simulink model "Modified_singlephasevienna"  (R2024a)
settings: Solver=VariableStepAuto  StartTime=0.0  StopTime=5  RelTol=1e-3
libraries: spsVoltageMeasurementLib x11, spsDiodeLib x10, spsCurrentMeasurementLib x8, spsSeriesRLCBranchLib x7, spsMosfetLib x4, spsIdealSwitchLib x2, slpidlib x2, spsVariableResistorLib x2, spsACVoltageSourceLib x1, simulink_extras x1, spsIGBTLib x1, spsLinearTransformerLib x1
settings Model: Creator=DELL  LastModifiedBy=DELL

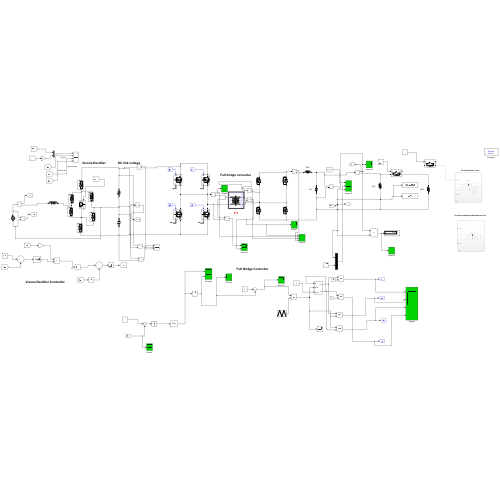
[thumbnail: Simulink's stored preview of the top-level diagram]
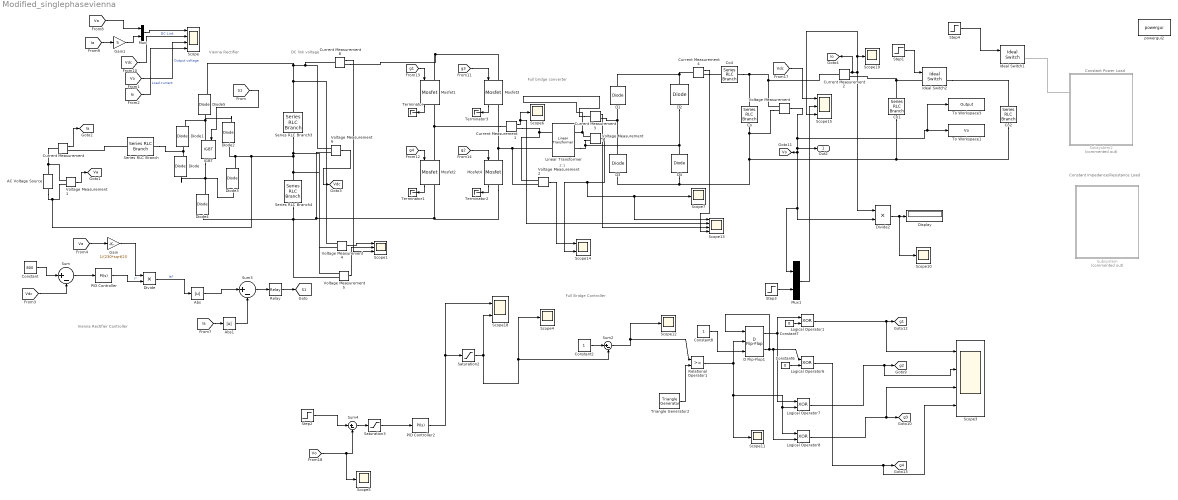
== system Modified_singlephasevienna ==
  note: Constant Power Load
  note: 2:1
  note: Full bridge converter
  note: Constant Impedance/Resistance Load
  note: Vienna Rectifier
  note: Vienna Rectifier Controller
  note: Full Bridge Controller
  note: DC link voltage
  AC Voltage Source : spsACVoltageSourceLib/AC Voltage Source  Amplitude=325  Phase=0  Frequency=50  SampleTime=0  Measurements=None  BusType=PV  Pref=10e3  Qref=0  Qmin=-inf  Qmax=+inf
  Abs : Abs  SaturateOnIntegerOverflow=off
  Abs1 : Abs  SaturateOnIntegerOverflow=off
  Co : spsSeriesRLCBranchLib/Series RLC Branch  LConnTagsString=__new0  RConnTagsString=__new0  BranchType=C  Resistance=1e-4  Inductance=200e-6  SetiL0=off  InitialCurrent=0  Capacitance=2000e-6  Setx0=off  InitialVoltage=24  Measurements=None
  Co1 : spsSeriesRLCBranchLib/Series RLC Branch  LConnTagsString=__new0  RConnTagsString=__new0  BranchType=R  Resistance=0.52  Inductance=200e-6  SetiL0=off  InitialCurrent=0  Capacitance=1000e-6  Setx0=off  InitialVoltage=24  Measurements=None
  Co2 : spsSeriesRLCBranchLib/Series RLC Branch  LConnTagsString=__new0  RConnTagsString=__new0  BranchType=R  Resistance=0.52  Inductance=200e-6  SetiL0=off  InitialCurrent=0  Capacitance=1000e-6  Setx0=off  InitialVoltage=24  Measurements=None
  Co4 : spsSeriesRLCBranchLib/Series RLC Branch  LConnTagsString=__new0  RConnTagsString=__new0  BranchType=L  Resistance=1e-4  Inductance=.01  SetiL0=off  InitialCurrent=0  Capacitance=1000e-6  Setx0=off  InitialVoltage=24  Measurements=None
  Constant : Constant  Value=800
  Constant2 : Constant
  Constant6 : Constant  Value=0
  Constant7 : Constant  Value=0
  Constant8 : Constant
  Current Measurement{,1..4,8} (6 alike) : spsCurrentMeasurementLib/Current Measurement  PhasorSimulation=off  OutputType=Complex  PSBequivalent=0
  D Flip-Flop1 : simulink_extras/Flip Flops/D Flip-Flop
  D{1..4} (4 alike) : spsDiodeLib/Diode  Ron=1e-3  Lon=0  Vf=0.5  IC=0  UseSnubber=off  Rs=1e6  Cs=inf  Measurements=off
  Diode{,1..5} (6 alike) : spsDiodeLib/Diode  Ron=0.001  Lon=0  Vf=0.8  IC=0  UseSnubber=0  Rs=500  Cs=250e-9  Measurements=on
  Display : Display
  Divide : Product  Inputs=**
  Divide2 : Product  Inputs=**
  Gain : Gain  Gain=1/(230*sqrt(2))
  Gain1 : Gain  Gain=5
  IGBT : spsIGBTLib/IGBT  Ron=0.001  Lon=0  Vf=1  Tf=1e-6  Tt=2e-6  IC=0  Rs=1e5  Cs=inf  Measurements=on
  Ideal Switch1 : spsIdealSwitchLib/Ideal Switch  Ron=0.001  Lon=0  IC=0  Rs=1e5  Cs=inf  Measurements=on
  Ideal Switch2 : spsIdealSwitchLib/Ideal Switch  Ron=0.001  Lon=0  IC=0  Rs=1e5  Cs=inf  Measurements=on
  Linear Transformer : spsLinearTransformerLib/Linear Transformer  UNITS=SI  NominalPower=[3000 10e3 ]  winding1="[200   1e-2  100e-6]"  winding2="[100  1e-2  1.36e-6 ]"  ThreeWindings=off  winding3=[50 1e-2 1.36e-6]  RmLm=[10e3 0.01]  Measurements=None  DataType=on
  Logical Operator{1,6..8} (4 alike) : Logic  Operator=XOR  AllPortsSameDT=off  OutDataTypeStr=boolean
  Mosfet{1..4} (4 alike) : spsMosfetLib/Mosfet  Ron=1e-3  Lon=0  Rd=1e-3  Vfd=0  IC=0  Rs=1e6  Cs=inf  Measurements=on
  Mux : Mux  Inputs=2
  Mux1 : Mux  Inputs=2
  PID Controller : slpidlib/PID Controller  Controller=PI  Form=Parallel  TimeDomain=Continuous-time  UseExternalTs=off  SampleTime=50e-6  IntegratorMethod=Forward Euler  FilterMethod=Forward Euler  ControllerParametersSource=internal  P=5  I=100  UseKiTs=off  D=0  UseExternalDerivativeSource=off  N=100  UseFilter=on  TunerSelectOption=Transfer Function Based (PID Tuner App)  InitialConditionSource=internal  InitialConditionForIntegrator=0  InitialConditionForFilter=0  DifferentiatorICPrevScaledInput=0  ExternalReset=none  TrackingMode=off  Kt=1  LimitOutput=on  SatLimitsSource=internal  UpperSaturationLimit=30  LowerSaturationLimit=0  LinearizeAsGain=on  AntiWindupMode=none  Kb=1  LimitIntegrator=off  UpperIntegratorSaturationLimit=inf  LowerIntegratorSaturationLimit=-inf  POutMin=[]  POutMax=[]  IOutMin=[]  IOutMax=[]  DOutMin=[]  DOutMax=[]  NOutMin=[]  NOutMax=[]  SumOutMin=[]  SumOutMax=[]  SaturationOutMin=[]  SaturationOutMax=[]  PParamMin=[]  PParamMax=[]  IParamMin=[]  IParamMax=[]  DParamMin=[]  DParamMax=[]  NParamMin=[]  NParamMax=[]  KbParamMin=[]  KbParamMax=[]  KtParamMin=[]  KtParamMax=[]  KbOutMin=[]  KbOutMax=[]  KtOutMin=[]  KtOutMax=[]  IntegratorOutMin=[]  IntegratorOutMax=[]  FilterOutMin=[]  FilterOutMax=[]  SumI1OutMin=[]  SumI1OutMax=[]  SumI2OutMin=[]  SumI2OutMax=[]  SumI3OutMin=[]  SumI3OutMax=[]  SumI4OutMin=[]  SumI4OutMax=[]  SumDOutMin=[]  SumDOutMax=[]  DifferentiatorOutMin=[]  DifferentiatorOutMax=[]  FilterDiffOutCoefMin=[]  FilterDiffOutCoefMax=[]  ReciprocalOutMin=[]  ReciprocalOutMax=[]  SumDenOutMin=[]  SumDenOutMax=[]  SumNumOutMin=[]  SumNumOutMax=[]  DivideOutMin=[]  DivideOutMax=[]  UdiffTsProdOutMin=[]  UdiffTsProdOutMax=[]  NTsProdOutMin=[]  NTsProdOutMax=[]  UintegralTsProdOutMin=[]  UintegralTsProdOutMax=[]  UngainTsProdOutMin=[]  UngainTsProdOutMax=[]  ClampingZeroOutDataTypeStr=Inherit: Inherit via back propagation  ClampingZeroOutMin=[]  ClampingZeroOutMax=[]  FilterDenConstantOutDataTypeStr=Inherit: Inherit via back propagation  FilterDenConstantOutMin=[]  FilterDenConstantOutMax=[]  PCopyOutDataTypeStr=Inherit: Inherit via back propagation  PCopyOutMin=[]  PCopyOutMax=[]  NCopyOutDataTypeStr=Inherit: Inherit via back propagation  NCopyOutMin=[]  NCopyOutMax=[]  IntegratorContinuousStateAttributes=''  IntegratorStateMustResolveToSignalObject=off  IntegratorRTWStateStorageClass=Auto  FilterContinuousStateAttributes=''  FilterStateMustResolveToSignalObject=off  FilterRTWStateStorageClass=Auto  ParallelPVariant=InternalParameters  IdealPVariant=Disabled  IVariant=InternalParameters  DVariant=Disabled  IntegratorVariant=Continuous  SatVariant=Enabled  AWVariant=Passthrough  PCopyVariant=Disabled  TRVariant=Disabled  FdbkBlocksVariant=Forward  IdealPFdbkVariant=Disabled  SatFdbkVariant=Disabled  DerivativeFilterVariant=Disabled  NVariant=Disabled  NCopyVariant=Disabled_SignalSpec  FilterICVariant=Disabled  IntegratorICVariant=InternalICs  ExternalResetVariant=Disabled  TRSumVariant=Passthrough  SumFdbkVariant=Disabled  SumVariant=Sum_PI  TsampFilterVariant=InternalTs  TsampNgainVariant=Passthrough  TsampIntegralVariant=Disabled_SignalSpec  ExternalSaturationOutDataTypeStr=Inherit: Same as second input  DerivativeSourceVariant=Disabled
  PID Controller2 : slpidlib/PID Controller  Controller=PI  Form=Parallel  TimeDomain=Continuous-time  UseExternalTs=off  SampleTime=-1  IntegratorMethod=Forward Euler  FilterMethod=Forward Euler  ControllerParametersSource=internal  P=1000  I=400  UseKiTs=off  D=3  UseExternalDerivativeSource=off  N=100  UseFilter=on  TunerSelectOption=Transfer Function Based (PID Tuner App)  InitialConditionSource=internal  InitialConditionForIntegrator=0  InitialConditionForFilter=0  DifferentiatorICPrevScaledInput=0  ExternalReset=none  TrackingMode=off  Kt=1  LimitOutput=off  SatLimitsSource=internal  UpperSaturationLimit=inf  LowerSaturationLimit=-inf  LinearizeAsGain=on  AntiWindupMode=none  Kb=1  LimitIntegrator=off  UpperIntegratorSaturationLimit=inf  LowerIntegratorSaturationLimit=-inf  POutMin=[]  POutMax=[]  IOutMin=[]  IOutMax=[]  DOutMin=[]  DOutMax=[]  NOutMin=[]  NOutMax=[]  SumOutMin=[]  SumOutMax=[]  SaturationOutMin=[]  SaturationOutMax=[]  PParamMin=[]  PParamMax=[]  IParamMin=[]  IParamMax=[]  DParamMin=[]  DParamMax=[]  NParamMin=[]  NParamMax=[]  KbParamMin=[]  KbParamMax=[]  KtParamMin=[]  KtParamMax=[]  KbOutMin=[]  KbOutMax=[]  KtOutMin=[]  KtOutMax=[]  IntegratorOutMin=[]  IntegratorOutMax=[]  FilterOutMin=[]  FilterOutMax=[]  SumI1OutMin=[]  SumI1OutMax=[]  SumI2OutMin=[]  SumI2OutMax=[]  SumI3OutMin=[]  SumI3OutMax=[]  SumI4OutMin=[]  SumI4OutMax=[]  SumDOutMin=[]  SumDOutMax=[]  DifferentiatorOutMin=[]  DifferentiatorOutMax=[]  FilterDiffOutCoefMin=[]  FilterDiffOutCoefMax=[]  ReciprocalOutMin=[]  ReciprocalOutMax=[]  SumDenOutMin=[]  SumDenOutMax=[]  SumNumOutMin=[]  SumNumOutMax=[]  DivideOutMin=[]  DivideOutMax=[]  UdiffTsProdOutMin=[]  UdiffTsProdOutMax=[]  NTsProdOutMin=[]  NTsProdOutMax=[]  UintegralTsProdOutMin=[]  UintegralTsProdOutMax=[]  UngainTsProdOutMin=[]  UngainTsProdOutMax=[]  ClampingZeroOutDataTypeStr=Inherit: Inherit via back propagation  ClampingZeroOutMin=[]  ClampingZeroOutMax=[]  FilterDenConstantOutDataTypeStr=Inherit: Inherit via back propagation  FilterDenConstantOutMin=[]  FilterDenConstantOutMax=[]  PCopyOutDataTypeStr=Inherit: Inherit via back propagation  PCopyOutMin=[]  PCopyOutMax=[]  NCopyOutDataTypeStr=Inherit: Inherit via back propagation  NCopyOutMin=[]  NCopyOutMax=[]  IntegratorContinuousStateAttributes=''  IntegratorStateMustResolveToSignalObject=off  IntegratorRTWStateStorageClass=Auto  FilterContinuousStateAttributes=''  FilterStateMustResolveToSignalObject=off  FilterRTWStateStorageClass=Auto  ParallelPVariant=InternalParameters  IdealPVariant=Disabled  IVariant=InternalParameters  DVariant=Disabled  IntegratorVariant=Continuous  SatVariant=Disabled  AWVariant=Passthrough  PCopyVariant=Disabled  TRVariant=Disabled  FdbkBlocksVariant=Forward  IdealPFdbkVariant=Disabled  SatFdbkVariant=Disabled  DerivativeFilterVariant=Disabled  NVariant=Disabled  NCopyVariant=Disabled_SignalSpec  FilterICVariant=Disabled  IntegratorICVariant=InternalICs  ExternalResetVariant=Disabled  TRSumVariant=Passthrough  SumFdbkVariant=Disabled  SumVariant=Sum_PI  TsampFilterVariant=InternalTs  TsampNgainVariant=Passthrough  TsampIntegralVariant=Disabled_SignalSpec  ExternalSaturationOutDataTypeStr=Inherit: Same as second input  DerivativeSourceVariant=Disabled
  Relational Operator1 : RelationalOperator  OutDataTypeStr=boolean  RndMeth=Floor  InputSameDT=off
  Relay : Relay
  Saturation2 : Saturate  UpperLimit=0.999  LowerLimit=0.001
  Saturation3 : Saturate  UpperLimit=0.1  LowerLimit=-100  LinearizeAsGain=off
  Scope : Scope  NumInputPorts=4
  Scope1 : Scope  NumInputPorts=3
  Scope{4..7,10..12,19} (8 alike) : Scope
  Scope13 : Scope  NumInputPorts=4
  Scope14 : Scope  NumInputPorts=2
  Scope15 : Scope  NumInputPorts=3
  Scope18 : Scope  NumInputPorts=2
  Scope3 : Scope  NumInputPorts=4
  Series RLC Branch : spsSeriesRLCBranchLib/Series RLC Branch  LConnTagsString=__new0  RConnTagsString=__new0  BranchType=L  Resistance=1  Inductance=1e-3  SetiL0=off  InitialCurrent=0  Capacitance=1e-6  Setx0=off  InitialVoltage=0  Measurements=None
  Series RLC Branch3 : spsSeriesRLCBranchLib/Series RLC Branch  LConnTagsString=__new0  RConnTagsString=__new0  BranchType=C  Resistance=1  Inductance=0.3e-3  SetiL0=off  InitialCurrent=0  Capacitance=750e-6  Setx0=off  InitialVoltage=0  Measurements=None
  Series RLC Branch4 : spsSeriesRLCBranchLib/Series RLC Branch  LConnTagsString=__new0  RConnTagsString=__new0  BranchType=C  Resistance=1  Inductance=0.3e-3  SetiL0=off  InitialCurrent=0  Capacitance=750e-6  Setx0=off  InitialVoltage=0  Measurements=None
  Step1 : Step  Time=2.5  SampleTime=0
  Step2 : Step  Time=5  Before=48  After=48  SampleTime=0
  Step3 : Step  Time=5  Before=48  After=48  SampleTime=0
  Step4 : Step  Time=0.6  SampleTime=0
  Subsystem : Subsystem  Commented=on
  Subsystem2 : Subsystem  Commented=on
  Sum{,2..4} (4 alike) : Sum  Inputs=|+-
  Terminator{,1..3} (4 alike) : Terminator
  To Workspace1 : ToWorkspace  VariableName=Vo  SaveFormat=Timeseries  SampleTime=-1
  To Workspace3 : ToWorkspace  VariableName=Output  SaveFormat=Timeseries  SampleTime=-1
  Triangle Generator2 : spsTriangleGeneratorLib/Triangle Generator  Freq=5000  Phase=0  Ts=0
  Voltage Measurement{,1..6} (7 alike) : spsVoltageMeasurementLib/Voltage Measurement  PhasorSimulation=off  OutputType=Complex  PSBequivalent=0
  powergui2 : spspowerguiLib/powergui  Priority=1  SimulationMode=Discrete  SampleTime=5e-6  frequency=60  Iterations=50  frequencyindice=0  Pbase=100e6  ErrMax=1e-4  UnitsV=kV  UnitsW=MW  buscounter=0  FunctionMessages=off  echomessages=off  EnableUseOfTLC=off  CurrentSourceSwitches=off  DisableSnubberDevices=off  DisableRonSwitches=off  DisableVfSwitches=off  DisplayEquations=off  AutomaticDiscreteSolvers=off  SolverType=Tustin/Backward Euler (TBE)  Interpol=off  ExternalGateDelay=off  methode=off  Ts=100  x0status=blocks  SPID=on  SwTol=0  HookPort=off  NonlinearTolerance=1e-4  nMaxIteration=100  ContinueOnMaxIteration=off  RestoreLinks=warning  ResistiveCurrentMeasurement=off  Frange=[0:2:500]  Ylog=off  Xlog=on  ShowGrid=off  save=off  variable=ZData  structure=0  ZoomFFT=off  StartTime=0.0  cycles=1  DisplayStyle=1  fundamental=60  FreqAxis=off  MaxFrequency=1000  frequencyindicesteady=1  RmsSteady=1  display=off
  Out2 : Outport
  tag scope: Ia=global, Io=global, S1=global, Va=global, Vdc=global, Vo=global, g1=global, g2=global, g3=global, g4=global
  wires:
  Voltage Measurement1/1 -> [Va]
  Current Measurement/1 -> [Ia]
  [Ia] -> Gain1/1
  [S1] -> IGBT/1
  Voltage Measurement6/1 -> [Vdc]
  [Ia] -> Abs1/1
  [Va] -> Gain/1
  Divide/1 -> Abs/1  "Ia*"
  Relay/1 -> [S1]
  Sum/1 -> PID Controller/1
  Abs1/1 -> Sum3/2
  Abs/1 -> Sum3/1
  Constant/1 -> Sum/1
  PID Controller/1 -> Divide/2  "I^"
  [Vdc] -> Sum/2
  Sum3/1 -> Relay/1
  Gain/1 -> Divide/1
  [Va] -> Mux/1
  Gain1/1 -> Mux/2
  Mux/1 -> Scope/1
  [g4] -> Mosfet2/1
  Current Measurement3/1 -> Scope13/3
  Saturation3/1 -> PID Controller2/1
  Current Measurement2/1 -> [Io], Scope15/3, Scope19/1, Divide2/1
  Constant6/1 -> Logical Operator6/2
  Divide2/1 -> Scope10/1, Display/1
  Step4/1 -> Ideal Switch1/1
  Constant2/1 -> Sum2/1
  PID Controller2/1 -> Saturation2/1, Scope18/1
  Logical Operator6/1 -> Scope3/4, [g4]
  Sum2/1 -> Scope12/1, Relational Operator1/1
  Mosfet2/1 -> Terminator1/1
  Step2/1 -> Sum4/1
  [g1] -> Mosfet1/1
  [Vo] -> Scope5/1, Sum4/2
  [Vdc] -> Scope15/1
  Logical Operator7/1 -> Scope3/2, [g2]
  Step3/1 -> Mux1/2
  Constant7/1 -> Logical Operator1/2
  Constant8/1 -> D Flip-Flop1/3
  Mosfet4/1 -> Terminator2/1
  Voltage Measurement3/1 -> Scope14/2, Scope13/1, Scope7/1
  Logical Operator1/1 -> Scope3/1, [g1]
  Voltage Measurement/1 -> Divide2/2, Mux1/1, [Vo], Out2/1, To Workspace3/1, To Workspace1/1
  D Flip-Flop1/1 -> Logical Operator7/1, Logical Operator1/1
  Sum4/1 -> Saturation3/1
  Mux1/1 -> Scope15/2
  Mosfet1/1 -> Terminator/1
  Current Measurement4/1 -> Scope13/4
  Mosfet3/1 -> Terminator3/1
  [g2] -> Mosfet4/1
  Relational Operator1/1 -> Logical Operator7/2, Logical Operator8/1, Scope11/1, D Flip-Flop1/2
  Current Measurement1/1 -> Scope13/2, Scope6/1
  Triangle Generator2/1 -> Relational Operator1/2
  Saturation2/1 -> Sum2/2, Scope4/1, Scope18/2
  [g3] -> Mosfet3/1
  Voltage Measurement2/1 -> Scope14/1
  Logical Operator8/1 -> Scope3/3, [g3]
  D Flip-Flop1/2 -> D Flip-Flop1/1, Logical Operator8/2, Logical Operator6/1
  [Vdc] -> Scope/2  "DC Link"
  [Vo] -> Scope/3  "Output voltage"
  [Io] -> Scope/4  "Load current"
  Voltage Measurement4/1 -> Scope1/1
  Voltage Measurement5/1 -> Scope1/2
  Current Measurement8/1 -> Scope1/3
  Step1/1 -> Ideal Switch2/1
  connections:
  IGBT/RConn1 -- Diode4/RConn1 -- Diode/LConn1 -- Diode3/LConn1
  Series RLC Branch3/LConn1 -- Voltage Measurement4/LConn1 -- Current Measurement8/LConn1 -- Voltage Measurement6/LConn1 -- Diode5/RConn1
  Diode1/LConn1 -- Series RLC Branch/RConn1 -- Diode/RConn1
  Diode5/LConn1 -- Diode2/RConn1 -- IGBT/LConn1 -- Diode1/RConn1
  Series RLC Branch/LConn1 -- Current Measurement/RConn1
  Series RLC Branch3/RConn1 -- Voltage Measurement4/LConn2 -- Voltage Measurement5/LConn1 -- Series RLC Branch4/LConn1 -- Diode2/LConn1 -- Diode3/RConn1 -- AC Voltage Source/LConn1 -- Voltage Measurement1/LConn2
  AC Voltage Source/RConn1 -- Voltage Measurement1/LConn1 -- Current Measurement/LConn1
  Co1/LConn1 -- Current Measurement2/RConn1 -- Ideal Switch2/LConn1
  Current Measurement3/RConn1 -- D1/LConn1 -- D3/RConn1
  Co4/LConn1 -- Co/LConn1 -- Voltage Measurement/LConn1 -- Current Measurement2/LConn1
  Voltage Measurement2/LConn1 -- Linear Transformer/LConn1 -- Current Measurement1/RConn1
  Current Measurement1/LConn1 -- Mosfet1/RConn1 -- Mosfet2/LConn1
  Current Measurement4/LConn1 -- D1/RConn1 -- D2/RConn1
  Mosfet3/LConn1 -- Current Measurement8/RConn1 -- Mosfet1/LConn1
  Mosfet4/LConn1 -- Mosfet3/RConn1 -- Linear Transformer/LConn2 -- Voltage Measurement2/LConn2
  Linear Transformer/RConn2 -- Voltage Measurement3/LConn2 -- D2/LConn1 -- D4/RConn1
  Current Measurement3/LConn1 -- Linear Transformer/RConn1 -- Voltage Measurement3/LConn1
  Voltage Measurement/LConn2 -- Co2/RConn1 -- Co1/RConn1 -- D4/LConn1 -- D3/LConn1 -- Co/RConn1
  Current Measurement4/RConn1 -- Co4/RConn1
  Series RLC Branch4/RConn1 -- Voltage Measurement6/LConn2 -- Mosfet2/RConn1 -- Mosfet4/RConn1 -- Voltage Measurement5/LConn2 -- Diode4/LConn1
  Subsystem2/LConn1 -- Ideal Switch1/RConn1
  Ideal Switch2/RConn1 -- Co2/LConn1

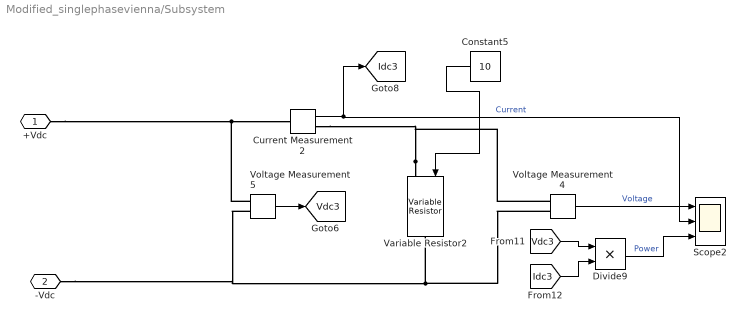
== system Modified_singlephasevienna/Subsystem ==
  Constant5 : Constant  Value=10
  Current Measurement2 : spsCurrentMeasurementLib/Current Measurement  PhasorSimulation=off  OutputType=Complex  PSBequivalent=0
  Divide9 : Product  Inputs=**
  Scope2 : Scope  NumInputPorts=3
  Variable Resistor2 : spsVariableResistorLib/Variable Resistor  Rabsmin=1
      settings: LibrarySourceBlock=sps_lib/Passives/Variable Resistor
  Voltage Measurement4 : spsVoltageMeasurementLib/Voltage Measurement  PhasorSimulation=off  OutputType=Complex  PSBequivalent=0
  Voltage Measurement5 : spsVoltageMeasurementLib/Voltage Measurement  PhasorSimulation=off  OutputType=Complex  PSBequivalent=0
  +Vdc : PMIOPort  Side=Left
  -Vdc : PMIOPort  Port=2  Side=Left
  tag scope: Idc3=global, Vdc3=global
  wires:
  Constant5/1 -> Variable Resistor2/1
  [Vdc3] -> Divide9/1
  Current Measurement2/1 -> [Idc3], Scope2/2  "Current"
  [Idc3] -> Divide9/2
  Divide9/1 -> Scope2/3  "Power"
  Voltage Measurement5/1 -> [Vdc3]
  Voltage Measurement4/1 -> Scope2/1  "Voltage"
  connections:
  Voltage Measurement5/LConn1 -- Current Measurement2/LConn1 -- +Vdc/RConn1
  Variable Resistor2/LConn1 -- Current Measurement2/RConn1 -- Voltage Measurement4/LConn1
  Voltage Measurement4/LConn2 -- Variable Resistor2/RConn1 -- -Vdc/RConn1 -- Voltage Measurement5/LConn2

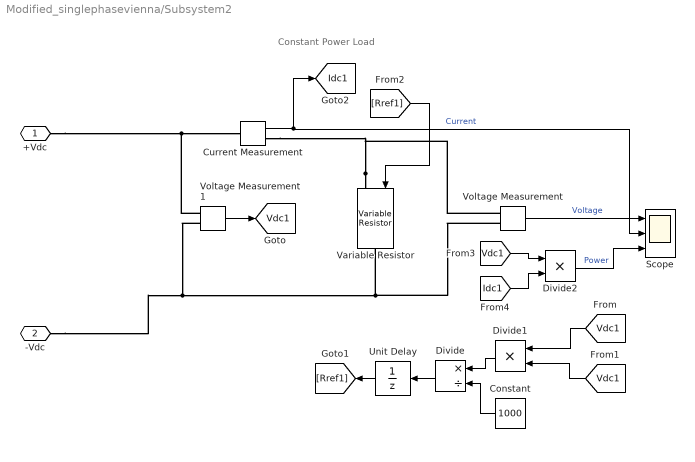
== system Modified_singlephasevienna/Subsystem2 ==
  note: Constant Power Load
  Constant : Constant  Value=1000
  Current Measurement : spsCurrentMeasurementLib/Current Measurement  PhasorSimulation=off  OutputType=Complex  PSBequivalent=0
  Divide : Product  Inputs=*/
  Divide1 : Product  Inputs=**
  Divide2 : Product  Inputs=**
  Scope : Scope  NumInputPorts=3
  Unit Delay : UnitDelay  SampleTime=5e-6  HasFrameUpgradeWarning=on
  Variable Resistor : spsVariableResistorLib/Variable Resistor  Rabsmin=1
      settings: LibrarySourceBlock=sps_lib/Passives/Variable Resistor
  Voltage Measurement : spsVoltageMeasurementLib/Voltage Measurement  PhasorSimulation=off  OutputType=Complex  PSBequivalent=0
  Voltage Measurement1 : spsVoltageMeasurementLib/Voltage Measurement  PhasorSimulation=off  OutputType=Complex  PSBequivalent=0
  +Vdc : PMIOPort  Side=Left
  -Vdc : PMIOPort  Port=2  Side=Left
  tag scope: Idc1=global, Vdc1=global
  wires:
  [Idc1] -> Divide2/2
  Current Measurement/1 -> [Idc1], Scope/2  "Current"
  Divide2/1 -> Scope/3  "Power"
  Divide/1 -> Unit Delay/1
  Voltage Measurement1/1 -> [Vdc1]
  Constant/1 -> Divide/2
  [Rref1] -> Variable Resistor/1
  [Vdc1] -> Divide1/2
  [Vdc1] -> Divide1/1
  Unit Delay/1 -> [Rref1]
  Voltage Measurement/1 -> Scope/1  "Voltage"
  [Vdc1] -> Divide2/1
  Divide1/1 -> Divide/1
  connections:
  Voltage Measurement1/LConn1 -- +Vdc/RConn1 -- Current Measurement/LConn1
  Voltage Measurement1/LConn2 -- -Vdc/RConn1 -- Voltage Measurement/LConn2 -- Variable Resistor/RConn1
  Variable Resistor/LConn1 -- Current Measurement/RConn1 -- Voltage Measurement/LConn1
